simulink model "sla_iir_sharing"  (R2015b)
settings: Solver=FixedStepDiscrete  SolverMode=SingleTasking  StartTime=0.0  StopTime=10.0  RelTol=1e-3
PreLoadFcn:
  | Hd = sla_iir_sharing_fdesign
  | Coeff1 = Hd.sosMatrix(1,:)
  | Coeff2 = Hd.sosMatrix(2,:)
libraries: simulink x1
settings Model: Creator=at-mt  LastModifiedBy=amatsumo
settings DataIOCC: SaveFormat=Array  SignalLoggingSaveFormat=ModelDataLogs  SaveOutput=off  SignalLogging=off  SaveTime=off
settings OptimizationCC: BlockReduction=off  ConditionallyExecuteInputs=off  DefaultParameterBehavior=Inlined  ExpressionDepthLimit=2147483647
settings DebuggingCC: AlgebraicLoopMsg=error  UnderspecifiedInitializationDetection=Classic  MergeDetectMultiDrivingBlocksExec=none  SolverPrmCheckMsg=warning  MultiTaskDSMMsg=warning  MultiTaskCondExecSysMsg=none  SingleTaskRateTransMsg=error  ParameterOverflowMsg=warning  FcnCallInpInsideContextMsg=UseLocalSettings  StateNameClashWarn=warning
settings HardwareCC: ProdBitPerPointer=32  ProdLargestAtomicFloat=None  ProdIntDivRoundTo=Undefined  ProdEndianess=Unspecified  ProdWordSize=32  ProdHWDeviceType=ASIC/FPGA->ASIC/FPGA  ProdEqTarget=off
settings GRTTargetCC: GeneratePreprocessorConditionals=Disable all  CombineOutputUpdateFcns=off  GRTInterface=on
settings ConfigComp: CovModelRefEnable=Off  CovSFcnEnable=off

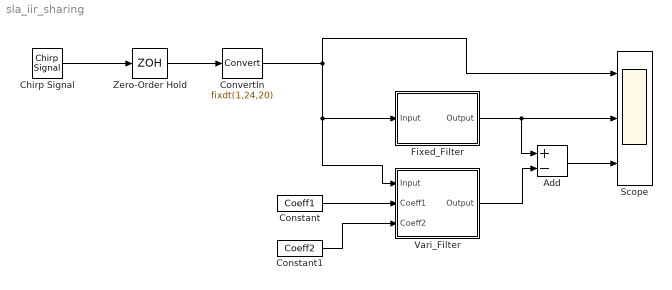
== system sla_iir_sharing ==
  Add : Sum  Inputs=+-
  Chirp Signal : simulink/Sources/Chirp Signal  f1=10  T=10  f2=500
  Constant : Constant  Value=Coeff1  OutDataTypeStr=fixdt(1,16,14)  SampleTime=-1
  Constant1 : Constant  Value=Coeff2  OutDataTypeStr=fixdt(1,16,14)  SampleTime=-1
  ConvertIn : DataTypeConversion  OutDataTypeStr=fixdt(1,24,20)  RndMeth=Nearest  SaturateOnIntegerOverflow=on
  Fixed_Filter : Subsystem  Tag=FilterWizardSubSystem
      settings: ErrorFcn=dspFilterRealizedInBasicElemsAlgLoopErrFcnCallback
  Scope : Scope  NumInputPorts=3
  Vari_Filter : Subsystem  Tag=FilterWizardSubSystem
      settings: ErrorFcn=dspFilterRealizedInBasicElemsAlgLoopErrFcnCallback
  Zero-Order Hold : ZeroOrderHold  SampleTime=1/1000
  wires:
  Zero-Order Hold/1 -> ConvertIn/1
  Chirp Signal/1 -> Zero-Order Hold/1
  Fixed_Filter/1(Output) -> Add/1, Scope/2
  ConvertIn/1 -> Vari_Filter/1(Input), Fixed_Filter/1(Input), Scope/1
  Vari_Filter/1(Output) -> Add/2
  Constant/1 -> Vari_Filter/2(Coeff1)
  Constant1/1 -> Vari_Filter/3(Coeff2)
  Add/1 -> Scope/3

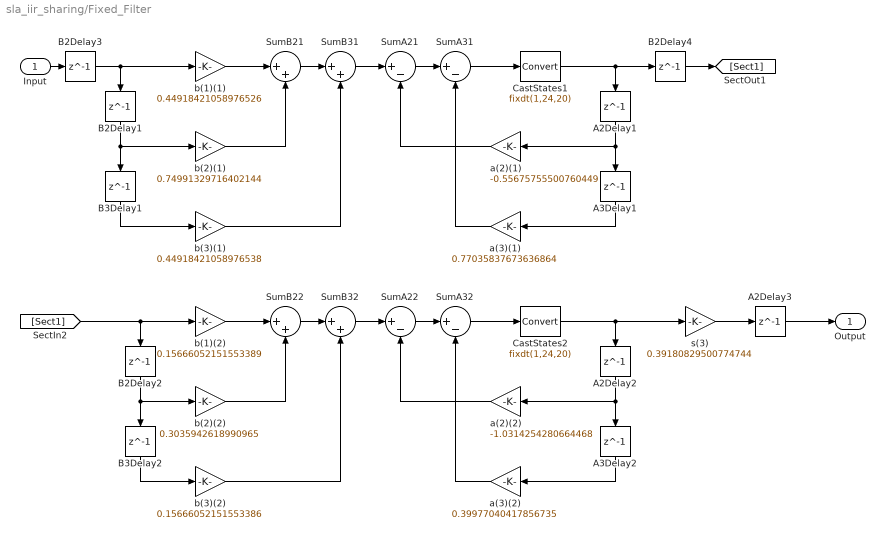
== system sla_iir_sharing/Fixed_Filter ==
  Input : Inport
  A2Delay1 : Delay  DelayLength=1  InitialCondition=0
  A2Delay2 : Delay  DelayLength=1  InitialCondition=0
  A2Delay3 : Delay  DelayLength=1  InitialCondition=0
  A3Delay1 : Delay  DelayLength=1  InitialCondition=0
  A3Delay2 : Delay  DelayLength=1  InitialCondition=0
  B2Delay{1..4} (4 alike) : Delay  DelayLength=1  InitialCondition=0
  B3Delay1 : Delay  DelayLength=1  InitialCondition=0
  B3Delay2 : Delay  DelayLength=1  InitialCondition=0
  CastStates1 : DataTypeConversion  OutDataTypeStr=fixdt(1,24,20)  RndMeth=Convergent
  CastStates2 : DataTypeConversion  OutDataTypeStr=fixdt(1,24,20)  RndMeth=Convergent
  SumA{21..22,31..32} (4 alike) : Sum  Inputs=|+-  AccumDataTypeStr=fixdt(1,40,34)  OutDataTypeStr=fixdt(1,40,34)  RndMeth=Convergent
  SumB{21..22,31..32} (4 alike) : Sum  Inputs=|++  AccumDataTypeStr=fixdt(1,40,35)  OutDataTypeStr=fixdt(1,40,35)  RndMeth=Convergent
  a(2)(1) : Gain  Gain=-0.55675755500760449  ParamDataTypeStr=fixdt(1,16,14)  OutDataTypeStr=fixdt(1,40,36)  RndMeth=Nearest
  a(2)(2) : Gain  Gain=-1.0314254280664468  ParamDataTypeStr=fixdt(1,16,14)  OutDataTypeStr=fixdt(1,40,36)  RndMeth=Nearest
  a(3)(1) : Gain  Gain=0.77035837673636864  ParamDataTypeStr=fixdt(1,16,14)  OutDataTypeStr=fixdt(1,40,36)  RndMeth=Nearest
  a(3)(2) : Gain  Gain=0.39977040417856735  ParamDataTypeStr=fixdt(1,16,14)  OutDataTypeStr=fixdt(1,40,36)  RndMeth=Nearest
  b(1)(1) : Gain  Gain=0.44918421058976526  ParamDataTypeStr=fixdt(1,16,14)  OutDataTypeStr=fixdt(1,40,36)  RndMeth=Nearest
  b(1)(2) : Gain  Gain=0.15666052151553389  ParamDataTypeStr=fixdt(1,16,14)  OutDataTypeStr=fixdt(1,40,36)  RndMeth=Nearest
  b(2)(1) : Gain  Gain=0.74991329716402144  ParamDataTypeStr=fixdt(1,16,14)  OutDataTypeStr=fixdt(1,40,36)  RndMeth=Nearest
  b(2)(2) : Gain  Gain=0.3035942618990965  ParamDataTypeStr=fixdt(1,16,14)  OutDataTypeStr=fixdt(1,40,36)  RndMeth=Nearest
  b(3)(1) : Gain  Gain=0.44918421058976538  ParamDataTypeStr=fixdt(1,16,14)  OutDataTypeStr=fixdt(1,40,36)  RndMeth=Nearest
  b(3)(2) : Gain  Gain=0.15666052151553386  ParamDataTypeStr=fixdt(1,16,14)  OutDataTypeStr=fixdt(1,40,36)  RndMeth=Nearest
  s(3) : Gain  Gain=0.39180829500774744  ParamDataTypeStr=fixdt(1,16,14)  OutDataTypeStr=fixdt(1,18,12)  RndMeth=Convergent
  Output : Outport
  wires:
  Input/1 -> B2Delay3/1
  b(1)(1)/1 -> SumB21/1
  SumB21/1 -> SumB31/1
  SumB31/1 -> SumA21/1
  SumA21/1 -> SumA31/1
  SumA31/1 -> CastStates1/1
  CastStates1/1 -> B2Delay4/1, A2Delay1/1
  B2Delay1/1 -> b(2)(1)/1, B3Delay1/1
  b(2)(1)/1 -> SumB21/2
  a(2)(1)/1 -> SumA21/2
  A2Delay1/1 -> a(2)(1)/1, A3Delay1/1
  B3Delay1/1 -> b(3)(1)/1
  b(3)(1)/1 -> SumB31/2
  a(3)(1)/1 -> SumA31/2
  A3Delay1/1 -> a(3)(1)/1
  [Sect1] -> b(1)(2)/1, B2Delay2/1
  b(1)(2)/1 -> SumB22/1
  SumB22/1 -> SumB32/1
  SumB32/1 -> SumA22/1
  SumA22/1 -> SumA32/1
  SumA32/1 -> CastStates2/1
  CastStates2/1 -> s(3)/1, A2Delay2/1
  B2Delay2/1 -> b(2)(2)/1, B3Delay2/1
  b(2)(2)/1 -> SumB22/2
  a(2)(2)/1 -> SumA22/2
  A2Delay2/1 -> a(2)(2)/1, A3Delay2/1
  B3Delay2/1 -> b(3)(2)/1
  b(3)(2)/1 -> SumB32/2
  a(3)(2)/1 -> SumA32/2
  A3Delay2/1 -> a(3)(2)/1
  s(3)/1 -> A2Delay3/1
  B2Delay3/1 -> b(1)(1)/1, B2Delay1/1
  B2Delay4/1 -> [Sect1]
  A2Delay3/1 -> Output/1

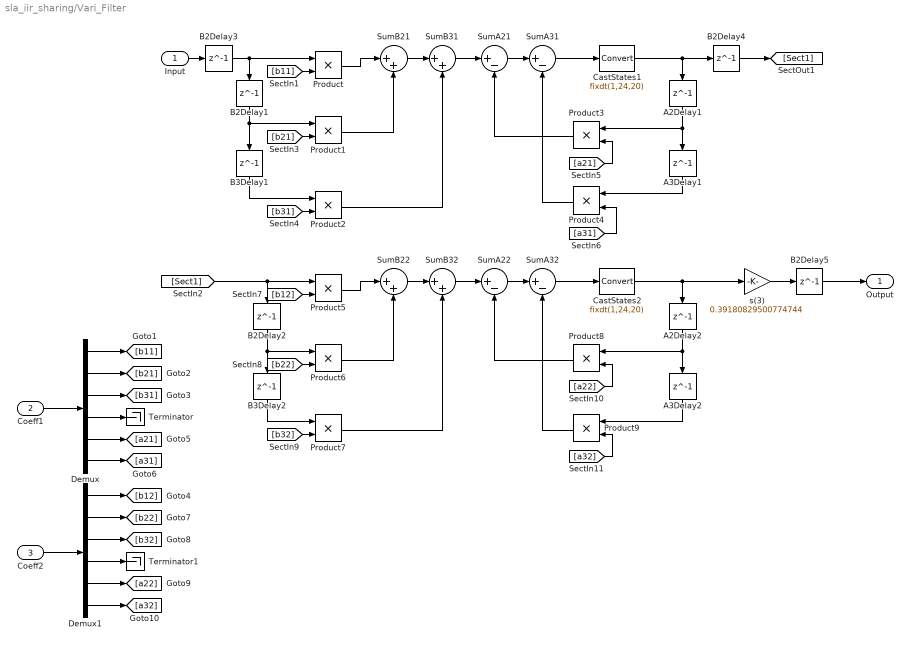
== system sla_iir_sharing/Vari_Filter ==
  Input : Inport
  Coeff1 : Inport  Port=2
  Coeff2 : Inport  Port=3
  A2Delay1 : Delay  DelayLength=1  InitialCondition=0
  A2Delay2 : Delay  DelayLength=1  InitialCondition=0
  A3Delay1 : Delay  DelayLength=1  InitialCondition=0
  A3Delay2 : Delay  DelayLength=1  InitialCondition=0
  B2Delay{1..5} (5 alike) : Delay  DelayLength=1  InitialCondition=0
  B3Delay1 : Delay  DelayLength=1  InitialCondition=0
  B3Delay2 : Delay  DelayLength=1  InitialCondition=0
  CastStates1 : DataTypeConversion  OutDataTypeStr=fixdt(1,24,20)  RndMeth=Convergent
  CastStates2 : DataTypeConversion  OutDataTypeStr=fixdt(1,24,20)  RndMeth=Convergent
  Demux : Demux  Outputs=6
  Demux1 : Demux  Outputs=6
  Product{,1..9} (10 alike) : Product  OutDataTypeStr=fixdt(1,40,36)  RndMeth=Nearest
  SumA{21..22,31..32} (4 alike) : Sum  Inputs=|+-  AccumDataTypeStr=fixdt(1,40,34)  OutDataTypeStr=fixdt(1,40,34)  RndMeth=Convergent
  SumB{21..22,31..32} (4 alike) : Sum  Inputs=|++  AccumDataTypeStr=fixdt(1,40,35)  OutDataTypeStr=fixdt(1,40,35)  RndMeth=Convergent
  Terminator : Terminator
  Terminator1 : Terminator
  s(3) : Gain  Gain=0.39180829500774744  ParamDataTypeStr=fixdt(1,16,14)  OutDataTypeStr=fixdt(1,18,12)  RndMeth=Convergent
  Output : Outport
  wires:
  Coeff1/1 -> Demux/1
  Demux/1 -> [b11]
  Input/1 -> B2Delay3/1
  Product/1 -> SumB21/1
  SumB21/1 -> SumB31/1
  SumB31/1 -> SumA21/1
  SumA21/1 -> SumA31/1
  SumA31/1 -> CastStates1/1
  CastStates1/1 -> B2Delay4/1, A2Delay1/1
  B2Delay1/1 -> B3Delay1/1, Product1/1
  Product1/1 -> SumB21/2
  Product3/1 -> SumA21/2
  A2Delay1/1 -> A3Delay1/1, Product3/1
  B3Delay1/1 -> Product2/1
  Product2/1 -> SumB31/2
  Product4/1 -> SumA31/2
  A3Delay1/1 -> Product4/1
  [Sect1] -> Product5/1, B2Delay2/1
  Product5/1 -> SumB22/1
  SumB22/1 -> SumB32/1
  SumB32/1 -> SumA22/1
  SumA22/1 -> SumA32/1
  SumA32/1 -> CastStates2/1
  CastStates2/1 -> s(3)/1, A2Delay2/1
  B2Delay2/1 -> B3Delay2/1, Product6/1
  Product6/1 -> SumB22/2
  Product8/1 -> SumA22/2
  A2Delay2/1 -> A3Delay2/1, Product8/1
  B3Delay2/1 -> Product7/1
  Product7/1 -> SumB32/2
  Product9/1 -> SumA32/2
  A3Delay2/1 -> Product9/1
  s(3)/1 -> B2Delay5/1
  Demux/2 -> [b21]
  Demux/3 -> [b31]
  Demux/4 -> Terminator/1
  Demux/5 -> [a21]
  Demux/6 -> [a31]
  Coeff2/1 -> Demux1/1
  Demux1/1 -> [b12]
  Demux1/2 -> [b22]
  Demux1/3 -> [b32]
  Demux1/4 -> Terminator1/1
  Demux1/5 -> [a22]
  Demux1/6 -> [a32]
  [b11] -> Product/2
  [b21] -> Product1/2
  [b31] -> Product2/2
  [a21] -> Product3/2
  [a31] -> Product4/2
  [b12] -> Product5/2
  [b22] -> Product6/2
  [b32] -> Product7/2
  [a22] -> Product8/2
  [a32] -> Product9/2
  B2Delay3/1 -> Product/1, B2Delay1/1
  B2Delay4/1 -> [Sect1]
  B2Delay5/1 -> Output/1
